simulink library "AMK_model_lib"  (R2022b)
settings: Solver=VariableStepAuto  StartTime=0.0  StopTime=10.0  RelTol=1e-3
libraries: dspstat3 x2, simulink x1
settings Model: Creator=dr_pa  LastModifiedBy=dr_pa

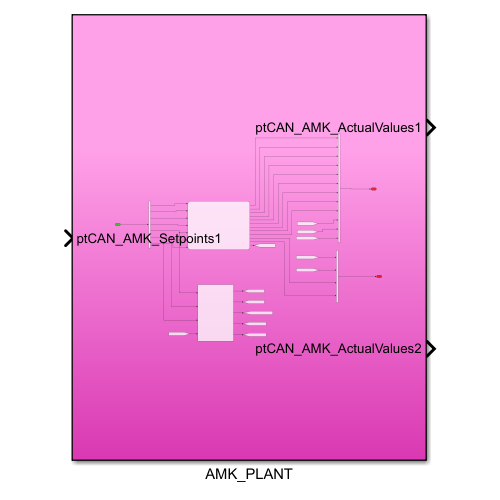
[thumbnail: Simulink's stored preview of the top-level diagram]
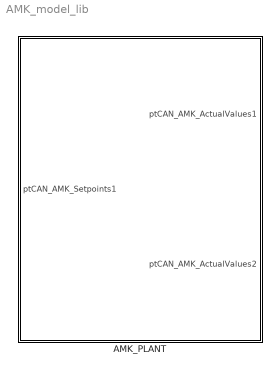
== system AMK_model_lib ==
  AMK_PLANT : Subsystem

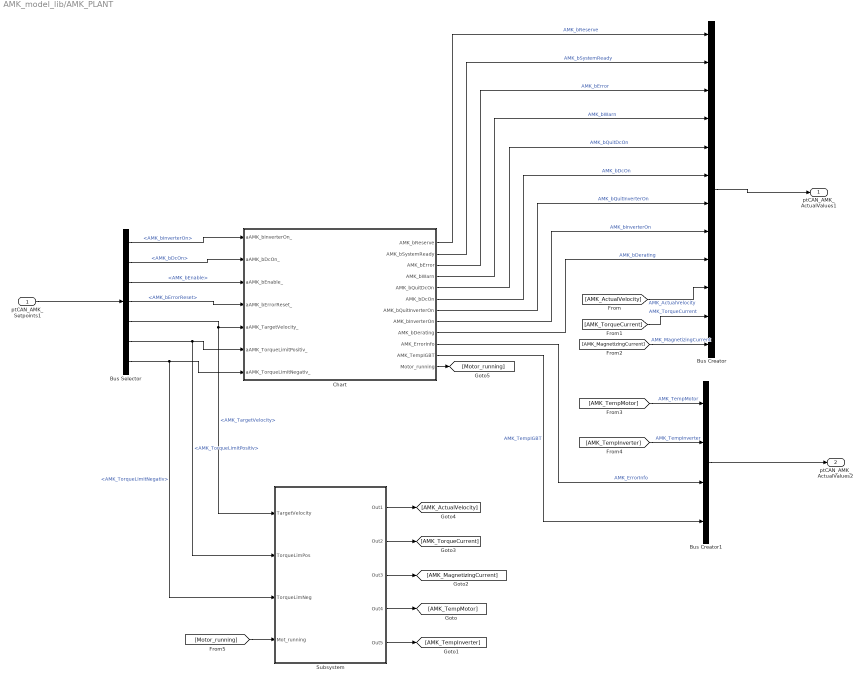
== system AMK_model_lib/AMK_PLANT ==
  ptCAN_AMK_Setpoints1 : Inport
  Bus Creator : BusCreator  Inputs=12
  Bus Creator1 : BusCreator  Inputs=4
  Bus Selector : BusSelector  OutputSignals=AMK_bInverterOn,AMK_bDcOn,AMK_bEnable,AMK_bErrorReset,AMK_TargetVelocity,AMK_TorqueLimitPositiv,AMK_TorqueLimitNegativ
  Chart : Stateflow chart  TreatAsAtomicUnit=on
  Subsystem : Subsystem
  ptCAN_AMK_ActualValues1 : Outport
  ptCAN_AMK_ActualValues2 : Outport  Port=2
  wires:
  Bus Creator/1 -> ptCAN_AMK_ActualValues1/1
  Chart/2(AMK_bSystemReady) -> Bus Creator/2  "AMK_bSystemReady"
  Chart/5(AMK_bQuitDcOn) -> Bus Creator/5  "AMK_bQuitDcOn"
  Chart/9(AMK_bDerating) -> Bus Creator/9  "AMK_bDerating"
  Chart/7(AMK_bQuitInverterOn) -> Bus Creator/7  "AMK_bQuitInverterOn"
  Chart/6(AMK_bDcOn) -> Bus Creator/6  "AMK_bDcOn"
  Chart/8(AMK_bInverterOn) -> Bus Creator/8  "AMK_bInverterOn"
  Chart/3(AMK_bError) -> Bus Creator/3  "AMK_bError"
  [AMK_ActualVelocity] -> Bus Creator/10  "AMK_ActualVelocity"
  Chart/4(AMK_bWarn) -> Bus Creator/4  "AMK_bWarn"
  [AMK_MagnetizingCurrent] -> Bus Creator/12  "AMK_MagnetizingCurrent"
  Chart/1(AMK_bReserve) -> Bus Creator/1  "AMK_bReserve"
  [AMK_TorqueCurrent] -> Bus Creator/11  "AMK_TorqueCurrent"
  Chart/10(AMK_ErrorInfo) -> Bus Creator1/3  "AMK_ErrorInfo"
  [AMK_TempInverter] -> Bus Creator1/2  "AMK_TempInverter"
  Chart/11(AMK_TempIGBT) -> Bus Creator1/4  "AMK_TempIGBT"
  [AMK_TempMotor] -> Bus Creator1/1  "AMK_TempMotor"
  Bus Creator1/1 -> ptCAN_AMK_ActualValues2/1
  ptCAN_AMK_Setpoints1/1 -> Bus Selector/1
  Bus Selector/1 -> Chart/1(aAMK_bInverterOn_)  "<AMK_bInverterOn>"
  Bus Selector/2 -> Chart/2(aAMK_bDcOn_)  "<AMK_bDcOn>"
  Bus Selector/3 -> Chart/3(aAMK_bEnable_)  "<AMK_bEnable>"
  Bus Selector/4 -> Chart/4(aAMK_bErrorReset_)  "<AMK_bErrorReset>"
  Bus Selector/5 -> Subsystem/1(TargetVelocity), Chart/5(aAMK_TargetVelocity_)  "<AMK_TargetVelocity>"
  Bus Selector/6 -> Subsystem/2(TorqueLimPos), Chart/6(aAMK_TorqueLimitPositiv_)  "<AMK_TorqueLimitPositiv>"
  Bus Selector/7 -> Subsystem/3(TorqueLimNeg), Chart/7(aAMK_TorqueLimitNegativ_)  "<AMK_TorqueLimitNegativ>"
  Chart/12(Motor_running) -> [Motor_running]
  [Motor_running] -> Subsystem/4(Mot_running)
  Subsystem/5(Out5) -> [AMK_TempInverter]
  Subsystem/4(Out4) -> [AMK_TempMotor]
  Subsystem/3(Out3) -> [AMK_MagnetizingCurrent]
  Subsystem/2(Out2) -> [AMK_TorqueCurrent]
  Subsystem/1(Out1) -> [AMK_ActualVelocity]

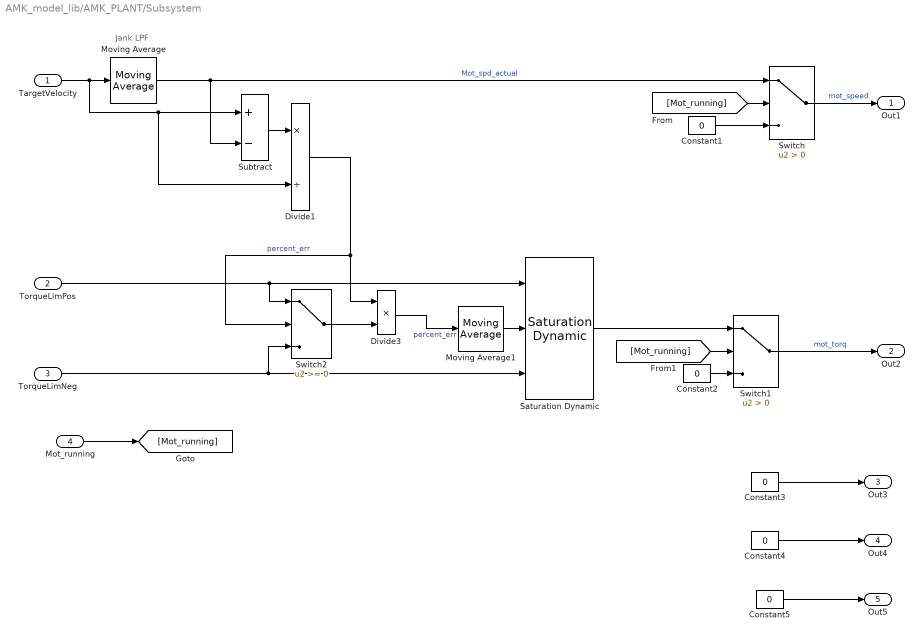
== system AMK_model_lib/AMK_PLANT/Subsystem ==
  note: Jank LPF
  TargetVelocity : Inport
  TorqueLimPos : Inport  Port=2
  TorqueLimNeg : Inport  Port=3
  Mot_running : Inport  Port=4
  Constant1 : Constant  Value=0
  Constant2 : Constant  Value=0
  Constant3 : Constant  Value=0  OutDataTypeStr=single
  Constant4 : Constant  Value=0  OutDataTypeStr=single
  Constant5 : Constant  Value=0  OutDataTypeStr=single
  Divide1 : Product  Inputs=*/
  Divide3 : Product  Inputs=**
  Moving Average : dspstat3/Moving Average  Method=Sliding window  ForgettingFactorPort=off  SpecifyWindowLength=on  WindowLength=10  OverlapLength=3  AllowArbitraryInputLength=off  ForgettingFactor=0.9  SimulateUsing=Code generation
  Moving Average1 : dspstat3/Moving Average  Method=Sliding window  ForgettingFactorPort=off  SpecifyWindowLength=on  WindowLength=3  OverlapLength=2  AllowArbitraryInputLength=off  ForgettingFactor=0.9  SimulateUsing=Code generation
  Saturation Dynamic : simulink/Discontinuities/Saturation Dynamic  OutMin=[]  OutMax=[]  OutDataTypeStr=Inherit: Same as second input  OutDataType=fixdt(1, 16)  OutScaling=2^-10  DoSatur=off
  Subtract : Sum  Inputs=+-
  Switch : Switch  Criteria=u2 > Threshold  OutDataTypeStr=single  SaturateOnIntegerOverflow=off  InputSameDT=off
  Switch1 : Switch  Criteria=u2 > Threshold  OutDataTypeStr=single  SaturateOnIntegerOverflow=off  InputSameDT=off
  Switch2 : Switch  SaturateOnIntegerOverflow=off  InputSameDT=off
  Out1 : Outport
  Out2 : Outport  Port=2
  Out3 : Outport  Port=3
  Out4 : Outport  Port=4
  Out5 : Outport  Port=5
  wires:
  Mot_running/1 -> [Mot_running]
  [Mot_running] -> Switch/2
  Switch/1 -> Out1/1  "mot_speed"
  Constant1/1 -> Switch/3
  Moving Average/1 -> Switch/1, Subtract/2  "Mot_spd_actual"
  Constant2/1 -> Switch1/3
  [Mot_running] -> Switch1/2
  Saturation Dynamic/1 -> Switch1/1
  Switch1/1 -> Out2/1  "mot_torq"
  Subtract/1 -> Divide1/1
  TargetVelocity/1 -> Divide1/2, Subtract/1, Moving Average/1
  Divide1/1 -> Divide3/1, Switch2/2  "percent_err"
  Constant3/1 -> Out3/1
  Constant4/1 -> Out4/1
  Constant5/1 -> Out5/1
  TorqueLimPos/1 -> Saturation Dynamic/1, Switch2/1
  Switch2/1 -> Divide3/2
  TorqueLimNeg/1 -> Switch2/3, Saturation Dynamic/3
  Moving Average1/1 -> Saturation Dynamic/2
  Divide3/1 -> Moving Average1/1  "percent_err"

== stateflow chart AMK_model_lib/AMK_PLANT/Chart ==
  state AMK_idle
    en:
    AMK_bReserve = 0;
    AMK_bSystemReady = 0;
    AMK_bError = 0;
    AMK_bWarn = 0;
    AMK_bQuitDcOn = 0;
    AMK_bDcOn = 0;
    AMK_bQuitInverterOn = 0;
    AMK_bInverterOn = 0;
    AMK_bDerating = 0;
    AMK_ActualVelocity = 0;
    AMK_TorqueCurrent = 0;
    AMK_MagnetizingCurrent = 0;
    Motor_running = false;
  note: Enable
      | en_
      | aAMK_bInverterOn_= 1
  state Startup [group]
    state Enable_System_Ready
      en:
      AMK_bSystemReady = 1;
    state Enable_Quit_Dc_On
      en:
      AMK_bQuitDcOn = 1;
      AMK_bDcOn = 1;
    state Inverter
    state bQuitDcOff
      en:
      AMK_bQuitDcOn = 0
    state Quit_Inventer_On
      en:
      AMK_bInverterOn = 1;
      AMK_bQuitInverterOn =1;
    state bDcOff
      en:
      AMK_bDcOn = 0
    state Inverter_Stuff2
      % (*3) and %(*4)
    state Motor_running
      en:
      Motor_running = true;
    state bEnable_off
      en:
      AMK_bQuitDcOn = 0
    state bInverter_off
      en:
      AMK_bInverterOn = 0
    state Inverter_Stuff1
      % (*6)
    state Shut_off_start
    Enable_System_Ready -> Enable_Quit_Dc_On : [aAMK_bDcOn_ == 1]
    Enable_Quit_Dc_On -> Inverter : [(abs(aAMK_TargetVelocity_) == 0) && ...
        | (abs(aAMK_TorqueLimitPositiv_) == 0) && ...
        | (abs(aAMK_TorqueLimitNegativ_) == 0)]
    Inverter -> Quit_Inventer_On : [(aAMK_bEnable_ == 1) && ...
        | (aAMK_bInverterOn_ == 1)]
    bDcOff -> bQuitDcOff
    Quit_Inventer_On -> Motor_running
    Inverter_Stuff2 -> bDcOff : [aAMK_bDcOn_ == 0]
    bEnable_off -> Inverter_Stuff2
    Motor_running -> Shut_off_start : [aAMK_TargetVelocity_ == 0 && aAMK_TorqueLimitPositiv_ == 0 && aAMK_TorqueLimitNegativ_ ==0]
    bInverter_off -> bEnable_off : [aAMK_bEnable_ == 0]
    Inverter_Stuff1 -> bInverter_off : [AMK_bInverterOn_ == 0]
    Shut_off_start -> Inverter_Stuff1
  (default) -> AMK_idle
  AMK_idle -> Enable_System_Ready : after(1,sec)
  data: aAMK_bInverterOn_ input; aAMK_bDcOn_ input; aAMK_bEnable_ input; aAMK_bErrorReset_ input; aAMK_TargetVelocity_ input; aAMK_TorqueLimitPositiv_ input; aAMK_TorqueLimitNegativ_ input; AMK_bReserve output boolean; AMK_bSystemReady output boolean; AMK_bError output boolean; AMK_bWarn output boolean; AMK_bQuitDcOn output boolean; AMK_bDcOn output boolean; AMK_bQuitInverterOn output boolean; AMK_bInverterOn output boolean; AMK_bDerating output boolean; AMK_ErrorInfo output int32; AMK_TempIGBT output single; Motor_running output boolean =false
